simulink model "Simulation3"  (R2024b)
settings: Solver=VariableStepAuto  StartTime=0.0  StopTime=30  RelTol=1e-3
libraries: vrlib x1
settings Model: Creator=alvinisac  LastModifiedBy=alvinisac

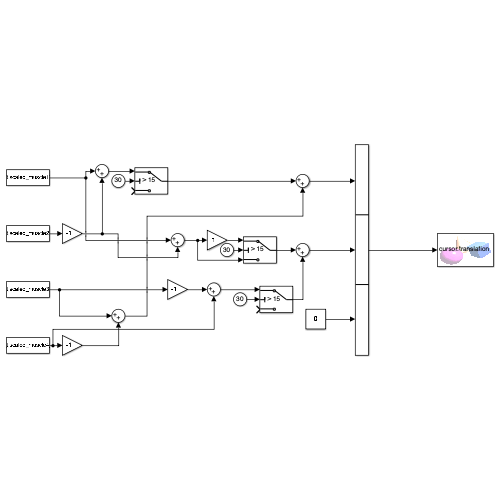
[thumbnail: Simulink's stored preview of the top-level diagram]
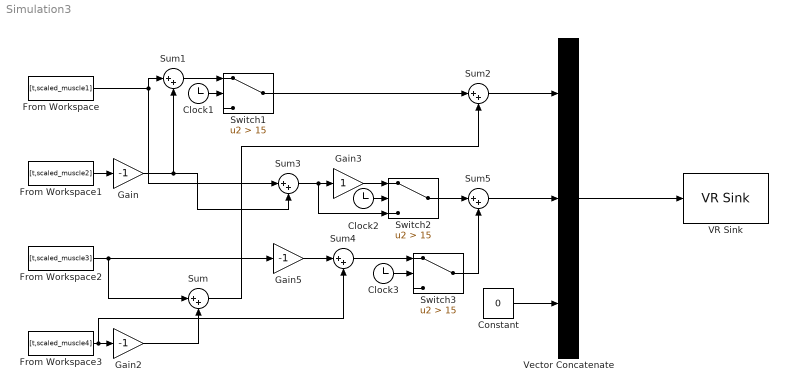
== system Simulation3 ==
  Clock1 : Clock
  Clock2 : Clock
  Clock3 : Clock
  Constant : Constant  Value=0
  From Workspace : FromWorkspace  VariableName=[t,scaled_muscle1]
  From Workspace1 : FromWorkspace  VariableName=[t,scaled_muscle2]
  From Workspace2 : FromWorkspace  VariableName=[t,scaled_muscle3]
  From Workspace3 : FromWorkspace  VariableName=[t,scaled_muscle4]
  Gain : Gain  Gain=-1
  Gain2 : Gain  Gain=-1
  Gain3 : Gain
  Gain5 : Gain  Gain=-1
  Sum{,1..5} (6 alike) : Sum  Inputs=|++
  Switch1 : Switch  Criteria=u2 > Threshold  Threshold=15  SaturateOnIntegerOverflow=off  InputSameDT=off
  Switch2 : Switch  Criteria=u2 > Threshold  Threshold=15  SaturateOnIntegerOverflow=off  InputSameDT=off
  Switch3 : Switch  Criteria=u2 > Threshold  Threshold=15  SaturateOnIntegerOverflow=off  InputSameDT=off
  VR Sink : vrlib/VR Sink  InstantiateOnLoad=on  SampleTime=0.1  ViewEnable=on  RemoteChange=off  RemoteView=off  FieldsWritten=cursor.translation.3.1.1.double  WorldFileName=8_palline_color.wrl  AutoView=off  VideoDimensions=[]  AllowVariableSize=off  FigureProperties="{'Position', 'Name', 'Viewpoint', 'CameraBound', 'CameraDirection', 'CameraPosition', 'CameraUpVector', 'ZoomFactor', 'Antialiasing', 'Headlight', 'Lighting', 'Sound', 'StatusBar', 'Stereo3D', 'Stereo3DCameraOffset', 'Stereo3DHIT', 'ToolBar', 'Textures', 'Transparency', 'Triad', 'Wireframe', 'NavZones', 'NavMode', 'NavSpeed', 'CaptureFileFormat', 'CaptureFileName', 'Record2DCompressMethod', 'Record2DCompressQuality', 'Record2D', 'Record2DFileName', 'Record2DFPS', 'NavPanel'; [5.0000000000000000e+00   1.0300000000000000e+02   5.7600000000000000e+02   3.5000000000000000e+02], '', '_untitled_1', 'on', [0.0000000000000000e+00   0.0000000000000000e+00  -1.0000000000000000e+00], [0.0000000000000000e+00   0.0000000000000000e+00   0.0000000000000000e+00], [0.0000000000000000e+00   1.0000000000000000e+00   0.0000000000000000e+00], [1.0000000000000000e+00], 'on', 'on', 'on', 'on', 'on', 'off', [1.0000000149011612e-01], [0.0000000000000000e+00], 'on', 'on', 'on', 'none', 'off', 'off', 'fly', 'normal', 'tif', '%f_anim_%n.tif', 'auto', [7.5000000000000000e+01], 'off', '%f_anim_%n.avi', 'auto', 'halfbar'}"
  Vector Concatenate : Concatenate  NumInputs=3
  wires:
  Vector Concatenate/1 -> VR Sink/1
  Gain2/1 -> Sum/2
  From Workspace2/1 -> Sum/1, Gain5/1
  From Workspace3/1 -> Sum4/2, Gain2/1
  Sum/1 -> Sum2/2
  Gain/1 -> Sum1/2, Sum3/2
  From Workspace/1 -> Sum3/1, Sum1/1
  From Workspace1/1 -> Gain/1
  Sum1/1 -> Switch1/1
  Clock1/1 -> Switch1/2
  Switch1/1 -> Sum2/1
  Sum2/1 -> Vector Concatenate/1
  Clock2/1 -> Switch2/2
  Sum3/1 -> Switch2/3, Gain3/1
  Switch2/1 -> Sum5/1
  Gain3/1 -> Switch2/1
  Gain5/1 -> Sum4/1
  Clock3/1 -> Switch3/2
  Sum4/1 -> Switch3/1
  Switch3/1 -> Sum5/2
  Sum5/1 -> Vector Concatenate/2
  Constant/1 -> Vector Concatenate/3
